simulink model "Fusion_Frame_Model_Architecture"  (R2018a)
settings: Solver=FixedStepAuto  StartTime=0.0  StopTime=SimulationTime  FixedStep=SamplingTime  RelTol=1e-3
undefined symbols (not defined in the file or in its folder): ACTIVATE_CAM, ACTIVATE_RAD, CAM1_detTimeStamp, CAM1_MeasNoise, CAM1_objClassID, CAM1_PX, CAM1_PY, CAM1_VX, CAM1_VY, CAM2_detTimeStamp, CAM2_MeasNoise, CAM2_objClassID, CAM2_PX, CAM2_PY, CAM2_VX, CAM2_VY, CAM3_detTimeStamp, CAM3_MeasNoise, CAM3_objClassID, CAM3_PX, CAM3_PY, CAM3_VX, CAM3_VY, CAM4_detTimeStamp, CAM4_MeasNoise, CAM4_objClassID, CAM4_PX, CAM4_PY, CAM4_VX, CAM4_VY, CAM5_detTimeStamp, CAM5_MeasNoise, CAM5_objClassID, CAM5_PX, CAM5_PY, CAM5_VX, CAM5_VY, CAM6_detTimeStamp, CAM6_MeasNoise, CAM6_objClassID, CAM6_PX, CAM6_PY, CAM6_VX, CAM6_VY, CAM7_detTimeStamp, CAM7_MeasNoise, CAM7_objClassID, CAM7_PX, CAM7_PY, CAM7_VX, CAM7_VY, CAM8_detTimeStamp, CAM8_MeasNoise, CAM8_objClassID, CAM8_PX, CAM8_PY, CAM8_VX, CAM8_VY, CAM_nMeas, CAM_TYPE ... (+181)
libraries: simulink_extras x4
(part 4 of 11)

== system Fusion_Frame_Model_Architecture/SENSOR_FUSION_SYSTEM/OBJECT_TRACKER_SENSOR_FUSION/SENSOR_LAYOUT_AND_CHRACTERIZATION/PRE_COMPUTE_SENSOR_FOV_GRID/SET_DATA ==
  GRID_PARAM : Inport
  RAD_REGION_CONFIDENCE : Inport  Port=2
  RAD_FOV_OVERLAP : Inport  Port=3
  CAM_REGION_CONFIDENCE : Inport  Port=4
  CAM_FOV_OVERLAP : Inport  Port=5
  Bus Creator : BusCreator  Inputs=2  OutDataTypeStr=Bus: RAD_GRID  NonVirtualBus=on
      settings: InheritFromInputs=off
  Bus Creator1 : BusCreator  Inputs=2  OutDataTypeStr=Bus: CAM_GRID  NonVirtualBus=on
      settings: InheritFromInputs=off
  Bus Creator2 : BusCreator  Inputs=3  OutDataTypeStr=Bus: GRID  NonVirtualBus=on
      settings: InheritFromInputs=off
  GRID_CHARACTERIZATION : Outport
  wires:
  Bus Creator/1 -> Bus Creator2/2  "RAD_GRID"
  CAM_REGION_CONFIDENCE/1 -> Bus Creator1/1  "CAM_REGION_CONFIDENCE"
  CAM_FOV_OVERLAP/1 -> Bus Creator1/2  "CAM_FOV_OVERLAP"
  Bus Creator1/1 -> Bus Creator2/3  "CAM_GRID"
  GRID_PARAM/1 -> Bus Creator2/1  "GRID_PARAM"
  RAD_REGION_CONFIDENCE/1 -> Bus Creator/1  "RAD_REGION_CONFIDENCE"
  RAD_FOV_OVERLAP/1 -> Bus Creator/2  "RAD_FOV_OVERLAP"
  Bus Creator2/1 -> GRID_CHARACTERIZATION/1

== system Fusion_Frame_Model_Architecture/SENSOR_FUSION_SYSTEM/OBJECT_TRACKER_SENSOR_FUSION/SENSOR_LAYOUT_AND_CHRACTERIZATION/SET_SENSOR_CALLIBRATION_PARAMETER/SET_CAMERA_SENSOR_PARAM ==
  CAMSnsrParam : Inport
  GET_DATA : Subsystem
  SET_CAMERA_EXTRINSIC_PARAM : Subsystem  TreatAsAtomicUnit=on
  SET_CAMERA_INTRINSIC_PARAM : Subsystem  TreatAsAtomicUnit=on
  SET_DATA : Subsystem
  CAMSnsrParamUpd : Outport
  wires:
  SET_DATA/1(CAMSnsrParamUpd) -> CAMSnsrParamUpd/1
  CAMSnsrParam/1 -> GET_DATA/1(CAMSnsrParam)
  GET_DATA/2(CameraExtrinsics) -> SET_CAMERA_EXTRINSIC_PARAM/1(CameraCalibParam)
  GET_DATA/1(CameraIntrinsics) -> SET_CAMERA_INTRINSIC_PARAM/1(CameraCalibParam)
  SET_CAMERA_INTRINSIC_PARAM/1(CameraCalibParamSet) -> SET_DATA/1(CameraIntrinsics)
  SET_CAMERA_EXTRINSIC_PARAM/1(CameraCalibParamSet) -> SET_DATA/2(CameraExtrinsics)

== system Fusion_Frame_Model_Architecture/SENSOR_FUSION_SYSTEM/OBJECT_TRACKER_SENSOR_FUSION/SENSOR_LAYOUT_AND_CHRACTERIZATION/SET_SENSOR_CALLIBRATION_PARAMETER/SET_RADAR_SENSOR_PARAM ==
  RADSnsrParam : Inport
  GET_DATA : Subsystem
  SET_DATA : Subsystem
  SET_RADAR_EXTRINSIC_PARAM : Subsystem  TreatAsAtomicUnit=on
  SET_RADAR_INTRINSIC_PARAM : Subsystem  TreatAsAtomicUnit=on
  RADSnsrParamUpd : Outport
  wires:
  RADSnsrParam/1 -> GET_DATA/1(RADSnsrParam)
  SET_DATA/1(RADSnsrParamUpd) -> RADSnsrParamUpd/1
  GET_DATA/2(<RadarExtrinsics>) -> SET_RADAR_EXTRINSIC_PARAM/1(RadarCalibParam)
  SET_RADAR_EXTRINSIC_PARAM/1(RadarCalibParamSet) -> SET_DATA/2(RadarExtrinsics)  "RadarIntrinsics"
  GET_DATA/1(<RadarIntrinsics>) -> SET_RADAR_INTRINSIC_PARAM/1(RadarCalibParam)
  SET_RADAR_INTRINSIC_PARAM/1(RadarCalibParamSet) -> SET_DATA/1(RadarIntrinsics)  "RadarExtrinsics"

== system Fusion_Frame_Model_Architecture/SENSOR_FUSION_SYSTEM/OBJECT_TRACKER_SENSOR_FUSION/SPATIAL_ALLIGNMENT1/CAMERA_MEASUREMENTS_SPATIAL_ALLIGNMENT/For Iterator Subsystem ==
  CameraCallibrationParam : Inport
  RadarStartingIdx : Inport  Port=2
  C1 : Inport  Port=3
  C2 : Inport  Port=4
  C3 : Inport  Port=5
  C4 : Inport  Port=6
  C5 : Inport  Port=7
  C6 : Inport  Port=8
  C7 : Inport  Port=9
  C8 : Inport  Port=10
  For Iterator : ForIterator  ResetStates=reset  IterationLimit=nCameras
  For Iterator Subsystem : Subsystem  TreatAsAtomicUnit=on
  InformationExtraction : Subsystem
  Subsystem : Subsystem
  MaxNoValidMeas : Outport
  CameraMeasTransformed : Outport  Port=2
  CameraMeasCOVTransformed : Outport  Port=3
  CameraMeasRef : Outport  Port=4
  wires:
  CameraCallibrationParam/1 -> InformationExtraction/1(CameraCallibration)
  C1/1 -> InformationExtraction/3(C1)
  C2/1 -> InformationExtraction/4(C2)
  C3/1 -> InformationExtraction/5(C3)
  C4/1 -> InformationExtraction/6(C4)
  C5/1 -> InformationExtraction/7(C5)
  C6/1 -> InformationExtraction/8(C6)
  InformationExtraction/1(CameraCalib) -> For Iterator Subsystem/1(CameraCalibration)
  InformationExtraction/2(nCameraMeas) -> For Iterator Subsystem/2(nMeas)
  InformationExtraction/3(CameraCANBus) -> For Iterator Subsystem/3(CameraCAN)
  RadarStartingIdx/1 -> InformationExtraction/11(StartingIndexes)
  Subsystem/1(nValidMeasVector) -> MaxNoValidMeas/1
  InformationExtraction/4(MeasStartingIdx) -> Subsystem/6(StartIdx)
  C7/1 -> InformationExtraction/9(C7)
  C8/1 -> InformationExtraction/10(C8)
  For Iterator/1 -> Subsystem/1(SnsrIndex), InformationExtraction/2(CameraID)
  For Iterator Subsystem/1(nValidMeas) -> Subsystem/2(nValidMeas)
  For Iterator Subsystem/2(CameraMeasUpd) -> Subsystem/3(CameraCTSMeas)
  For Iterator Subsystem/3(CameraMeasNoiseCovUpd) -> Subsystem/4(CameraCTSNoiseCOV)
  For Iterator Subsystem/4(CameraMeasRefUpd) -> Subsystem/5(CameraCTSRef)
  Subsystem/2(CTSMat) -> CameraMeasTransformed/1
  Subsystem/4(CTSMatRef) -> CameraMeasRef/1
  Subsystem/3(CTSMatNoiseCOV) -> CameraMeasCOVTransformed/1

== system Fusion_Frame_Model_Architecture/SENSOR_FUSION_SYSTEM/OBJECT_TRACKER_SENSOR_FUSION/SPATIAL_ALLIGNMENT1/CAMERA_MEASUREMENTS_SPATIAL_ALLIGNMENT/RadarMeasurementIndexes2 ==
  validMeasCount : Inport
  CTSmeasMAT : Inport  Port=2
  CTSCovMAT : Inport  Port=3
  CTSRefMAT : Inport  Port=4
  Add{,1..6} (7 alike) : Sum
  Assignment1 : Assignment  NumberOfDimensions=2  DiagnosticForDimensions=Warning  IndexOptions=Assign all,Starting index (dialog)  Indices=1,1  OutputSizes=1,1
  Assignment2 : Assignment  NumberOfDimensions=3  DiagnosticForDimensions=Warning  IndexOptions=Assign all,Assign all,Starting index (dialog)  Indices=1,1,1  OutputSizes=1,1,1
  Assignment3 : Assignment  NumberOfDimensions=2  DiagnosticForDimensions=Warning  IndexOptions=Assign all,Starting index (dialog)  Indices=1,1  OutputSizes=1,1
  Bus Creator1 : BusCreator  Inputs=5  OutDataTypeStr=Bus: CAM_MEAS_MAT_CTS  NonVirtualBus=on
      settings: InheritFromInputs=off
  FIND1 : Subsystem  TreatAsAtomicUnit=on
  Find Nonzero Elements1 : Find  Commented=on  NumberOfInputDimensions=3
  Mux1 : Mux  Inputs=8
  Reshape1 : Reshape  OutputDimensionality=Row vector (2-D)
  Selector : Selector  NumberOfDimensions=2  InputPortWidth=3  IndexOptions=Select all,Index vector (dialog)  Indices=1,1  OutputSizes=1,1
  Selector1 : Selector  NumberOfDimensions=2  InputPortWidth=3  IndexOptions=Select all,Index vector (dialog)  Indices=6,7  OutputSizes=1,1
  Selector11 : Selector  NumberOfDimensions=2  InputPortWidth=3  IndexOptions=Index vector (dialog),Select all  Indices=1,1  OutputSizes=1,1
  Selector12 : Selector  NumberOfDimensions=2  InputPortWidth=3  IndexOptions=Select all,Index vector (port)  Indices=1,1  OutputSizes=1,1
  Selector14 : Selector  NumberOfDimensions=2  InputPortWidth=3  IndexOptions=Select all,Index vector (port)  Indices=1,1  OutputSizes=1,1
  Selector15 : Selector  NumberOfDimensions=3  InputPortWidth=3  IndexOptions=Select all,Select all,Index vector (port)  Indices=1,1,1  OutputSizes=1,1,1
  Selector2 : Selector  NumberOfDimensions=2  InputPortWidth=3  IndexOptions=Select all,Index vector (dialog)  Indices=5,2  OutputSizes=1,1
  Selector3 : Selector  NumberOfDimensions=2  InputPortWidth=3  IndexOptions=Select all,Index vector (dialog)  Indices=5,3  OutputSizes=1,1
  Selector4 : Selector  NumberOfDimensions=2  InputPortWidth=3  IndexOptions=Select all,Index vector (dialog)  Indices=5,5  OutputSizes=1,1
  Selector5 : Selector  NumberOfDimensions=2  InputPortWidth=3  IndexOptions=Select all,Index vector (dialog)  Indices=6,6  OutputSizes=1,1
  Selector6 : Selector  NumberOfDimensions=2  InputPortWidth=3  IndexOptions=Select all,Index vector (dialog)  Indices=6,8  OutputSizes=1,1
  Selector8 : Selector  NumberOfDimensions=2  InputPortWidth=3  IndexOptions=Select all,Index vector (dialog)  Indices=5,4  OutputSizes=1,1
  CTSmeasMATout : Outport
  wires:
  validMeasCount/1 -> Selector2/1, Selector/1, Bus Creator1/4, Selector3/1, Selector6/1, Selector1/1, Selector5/1, Selector4/1, Selector8/1  "ValidMeasCountMeasCount"
  Add3/1 -> Add4/1, Mux1/5
  Selector3/1 -> Add1/2
  Add2/1 -> Add3/1, Mux1/4
  Add1/1 -> Mux1/3, Add2/1
  Selector4/1 -> Add3/2
  Selector/1 -> Mux1/1, Add/1
  Add/1 -> Add1/1, Mux1/2
  Add4/1 -> Add5/1, Mux1/6
  Selector2/1 -> Add/2
  Selector8/1 -> Add2/2
  Mux1/1 -> Reshape1/1
  Selector5/1 -> Add4/2
  Bus Creator1/1 -> CTSmeasMATout/1
  CTSRefMAT/1 -> [Ref], Selector11/1
  Selector11/1 -> FIND1/1(measIdx)
  FIND1/1(ValidIndex) -> Selector14/2, Selector12/2, Selector15/2
  CTSmeasMAT/1 -> Assignment1/1, Selector14/1
  Selector14/1 -> Assignment1/2
  Selector15/1 -> Assignment2/2
  Selector12/1 -> Assignment3/2
  CTSCovMAT/1 -> Assignment2/1, Selector15/1
  Assignment3/1 -> Bus Creator1/3  "MeasRef"
  Assignment2/1 -> Bus Creator1/2  "MeasCovariance"
  Assignment1/1 -> Bus Creator1/1  "MeasArray"
  [Ref] -> Assignment3/1, Selector12/1
  Reshape1/1 -> Bus Creator1/5  "ValidCumulativeMeasCount"
  Add5/1 -> Add6/1, Mux1/7
  Selector1/1 -> Add5/2
  Add6/1 -> Mux1/8
  Selector6/1 -> Add6/2

== system Fusion_Frame_Model_Architecture/SENSOR_FUSION_SYSTEM/OBJECT_TRACKER_SENSOR_FUSION/SPATIAL_ALLIGNMENT1/CAMERA_MEASUREMENTS_SPATIAL_ALLIGNMENT/StartingIndexes1 ==
  SnsrCallib : Inport
  CallibrationInfoExtractor : Subsystem
  Subsystem : Subsystem
  StartingIndexes : Outport
  wires:
  CallibrationInfoExtractor/1(C1nMeas) -> Subsystem/1(C1nMeas)
  CallibrationInfoExtractor/2(C2nMeas) -> Subsystem/2(C2nMeas)
  CallibrationInfoExtractor/3(C3nMeas) -> Subsystem/3(C3nMeas)
  CallibrationInfoExtractor/4(C4nMeas) -> Subsystem/4(C4nMeas)
  CallibrationInfoExtractor/5(C5nMeas) -> Subsystem/5(C5nMeas)
  Subsystem/1(StartingIndexes) -> StartingIndexes/1
  SnsrCallib/1 -> CallibrationInfoExtractor/1(SnsrCallib)
  CallibrationInfoExtractor/6(C6nMeas) -> Subsystem/6(C6nMeas)
  CallibrationInfoExtractor/7(C7nMeas) -> Subsystem/7(C7nMeas)

== system Fusion_Frame_Model_Architecture/SENSOR_FUSION_SYSTEM/OBJECT_TRACKER_SENSOR_FUSION/SPATIAL_ALLIGNMENT1/RADAR_MEASUREMENTS_SPATIAL_ALLIGNMENT/RADAR_MEASUREMENTS_SPATIAL_ALLIGNMENT ==
  RadarCallibrationParam : Inport
  RadarStartingIdx : Inport  Port=2
  R1 : Inport  Port=3
  R2 : Inport  Port=4
  R3 : Inport  Port=5
  R4 : Inport  Port=6
  R5 : Inport  Port=7
  R6 : Inport  Port=8
  COORDINATE_TRANSFORMATION : Subsystem  TreatAsAtomicUnit=on
  GET_DATA : Subsystem
  SENSOR_LOOP : ForIterator  ResetStates=reset  IterationLimit=nRadars
  SET_DATA : Subsystem
  RadarMeasTransformed : Outport
  RadarMeasCOVTransformed : Outport  Port=2
  RadarMeasRef : Outport  Port=3
  MaxNoValidMeas : Outport  Port=4
  wires:
  RadarCallibrationParam/1 -> GET_DATA/1(RadarCallibration)
  R1/1 -> GET_DATA/3(R1)
  R2/1 -> GET_DATA/4(R2)
  R3/1 -> GET_DATA/5(R3)
  R4/1 -> GET_DATA/6(R4)
  R5/1 -> GET_DATA/7(R5)
  R6/1 -> GET_DATA/8(R6)
  GET_DATA/1(RadarCalib) -> COORDINATE_TRANSFORMATION/1(RadarCalibration)
  GET_DATA/2(nRadarMeas) -> COORDINATE_TRANSFORMATION/2(nMeas)
  GET_DATA/3(RadarCANBus) -> COORDINATE_TRANSFORMATION/3(RadarCAN)
  RadarStartingIdx/1 -> GET_DATA/9(StartingIndexes)
  SENSOR_LOOP/1 -> SET_DATA/1(SnsrIndex), GET_DATA/2(RadarID)
  SET_DATA/1(nValidMeasVector) -> MaxNoValidMeas/1
  GET_DATA/4(MeasStartingIdx) -> SET_DATA/6(StartIdx)
  COORDINATE_TRANSFORMATION/1(nValidMeas) -> SET_DATA/2(nValidMeas)
  COORDINATE_TRANSFORMATION/2(RadarMeasUpd) -> SET_DATA/3(RadarCTSMeas)
  SET_DATA/2(CTSMat) -> RadarMeasTransformed/1
  COORDINATE_TRANSFORMATION/3(RadarMeasNoiseCovUpd) -> SET_DATA/4(RadarCTSNoiseCOV)
  COORDINATE_TRANSFORMATION/4(RadarMeasRefUpd) -> SET_DATA/5(RadarCTSRef)
  SET_DATA/4(CTSMatRef) -> RadarMeasRef/1
  SET_DATA/3(CTSMatNoiseCOV) -> RadarMeasCOVTransformed/1

== system Fusion_Frame_Model_Architecture/SENSOR_FUSION_SYSTEM/OBJECT_TRACKER_SENSOR_FUSION/SPATIAL_ALLIGNMENT1/RADAR_MEASUREMENTS_SPATIAL_ALLIGNMENT/SET_MEASUREMENTS ==
  CTSmeasMAT : Inport
  CTSCovMAT : Inport  Port=2
  CTSRefMAT : Inport  Port=3
  validMeasCount : Inport  Port=4
  Add{,1..4} (5 alike) : Sum
  Assignment1 : Assignment  NumberOfDimensions=2  DiagnosticForDimensions=Warning  IndexOptions=Assign all,Starting index (dialog)  Indices=1,1  OutputSizes=1,1
  Assignment2 : Assignment  NumberOfDimensions=3  DiagnosticForDimensions=Warning  IndexOptions=Assign all,Assign all,Starting index (dialog)  Indices=1,1,1  OutputSizes=1,1,1
  Assignment3 : Assignment  NumberOfDimensions=2  DiagnosticForDimensions=Warning  IndexOptions=Assign all,Starting index (dialog)  Indices=1,1  OutputSizes=1,1
  Bus Creator1 : BusCreator  Inputs=5  OutDataTypeStr=Bus: RAD_MEAS_MAT_CTS  NonVirtualBus=on
      settings: InheritFromInputs=off
  FIND : Subsystem  TreatAsAtomicUnit=on
  Find Nonzero Elements1 : Find  Commented=on  NumberOfInputDimensions=3
  Mux1 : Mux  Inputs=6
  Reshape1 : Reshape  OutputDimensionality=Row vector (2-D)
  Selector : Selector  NumberOfDimensions=2  InputPortWidth=3  IndexOptions=Select all,Index vector (dialog)  Indices=1,1  OutputSizes=1,1
  Selector11 : Selector  NumberOfDimensions=2  InputPortWidth=3  IndexOptions=Index vector (dialog),Select all  Indices=1,1  OutputSizes=1,1
  Selector12 : Selector  NumberOfDimensions=2  InputPortWidth=3  IndexOptions=Select all,Index vector (port)  Indices=1,1  OutputSizes=1,1
  Selector14 : Selector  NumberOfDimensions=2  InputPortWidth=3  IndexOptions=Select all,Index vector (port)  Indices=1,1  OutputSizes=1,1
  Selector15 : Selector  NumberOfDimensions=3  InputPortWidth=3  IndexOptions=Select all,Select all,Index vector (port)  Indices=1,1,1  OutputSizes=1,1,1
  Selector2 : Selector  NumberOfDimensions=2  InputPortWidth=3  IndexOptions=Select all,Index vector (dialog)  Indices=5,2  OutputSizes=1,1
  Selector3 : Selector  NumberOfDimensions=2  InputPortWidth=3  IndexOptions=Select all,Index vector (dialog)  Indices=5,3  OutputSizes=1,1
  Selector4 : Selector  NumberOfDimensions=2  InputPortWidth=3  IndexOptions=Select all,Index vector (dialog)  Indices=5,5  OutputSizes=1,1
  Selector5 : Selector  NumberOfDimensions=2  InputPortWidth=3  IndexOptions=Select all,Index vector (dialog)  Indices=6,6  OutputSizes=1,1
  Selector8 : Selector  NumberOfDimensions=2  InputPortWidth=3  IndexOptions=Select all,Index vector (dialog)  Indices=5,4  OutputSizes=1,1
  CTSmeasMATout : Outport
  wires:
  validMeasCount/1 -> Selector2/1, Selector/1, Bus Creator1/4, Selector3/1, Selector8/1, Selector4/1, Selector5/1  "ValidMeasCountMeasCount"
  Add3/1 -> Add4/1, Mux1/5
  Selector3/1 -> Add1/2
  Add2/1 -> Add3/1, Mux1/4
  Add1/1 -> Mux1/3, Add2/1
  Selector4/1 -> Add3/2
  Selector/1 -> Mux1/1, Add/1
  Add/1 -> Add1/1, Mux1/2
  Add4/1 -> Mux1/6
  Selector2/1 -> Add/2
  Selector8/1 -> Add2/2
  Mux1/1 -> Reshape1/1
  Selector5/1 -> Add4/2
  Bus Creator1/1 -> CTSmeasMATout/1
  CTSRefMAT/1 -> [Ref], Selector11/1
  Selector11/1 -> FIND/1(measIdx)
  FIND/1(ValidIndex) -> Selector14/2, Selector12/2, Selector15/2
  CTSmeasMAT/1 -> Assignment1/1, Selector14/1
  Selector14/1 -> Assignment1/2
  Selector15/1 -> Assignment2/2
  Selector12/1 -> Assignment3/2
  CTSCovMAT/1 -> Assignment2/1, Selector15/1
  Assignment3/1 -> Bus Creator1/3  "MeasRef"
  Assignment2/1 -> Bus Creator1/2  "MeasCovariance"
  Assignment1/1 -> Bus Creator1/1  "MeasArray"
  [Ref] -> Assignment3/1, Selector12/1
  Reshape1/1 -> Bus Creator1/5  "ValidCumulativeMeasCount"

== system Fusion_Frame_Model_Architecture/SENSOR_FUSION_SYSTEM/OBJECT_TRACKER_SENSOR_FUSION/SPATIAL_ALLIGNMENT1/RADAR_MEASUREMENTS_SPATIAL_ALLIGNMENT/StartingIndexes1 ==
  SnsrCallib : Inport
  CallibrationInfoExtractor : Subsystem
  Subsystem : Subsystem
  StartingIndexes : Outport
  wires:
  CallibrationInfoExtractor/1(R1nMeas) -> Subsystem/1(R1nMeas)
  CallibrationInfoExtractor/2(R2nMeas) -> Subsystem/2(R2nMeas)
  CallibrationInfoExtractor/3(R3nMeas) -> Subsystem/3(R3nMeas)
  CallibrationInfoExtractor/4(R4nMeas) -> Subsystem/4(R4nMeas)
  CallibrationInfoExtractor/5(R5nMeas) -> Subsystem/5(R5nMeas)
  Subsystem/1(StartingIndexes) -> StartingIndexes/1
  SnsrCallib/1 -> CallibrationInfoExtractor/1(SnsrCallib)

== system Fusion_Frame_Model_Architecture/SENSOR_FUSION_SYSTEM/ROAD_GEOMETRY_CAMERA_FUSION/ROAD_GEOMERY_AND_GRID_COMPUTATION/COMPUTE_LEFT_LINE/CURVE_FITTING_BY_LEAST_SQUARES ==
  Points : Inport
  Ground : Ground
  Terminator : Terminator
  PolynomialCoefficients : Outport
  wires:
  Points/1 -> Terminator/1
  Ground/1 -> PolynomialCoefficients/1

== system Fusion_Frame_Model_Architecture/SENSOR_FUSION_SYSTEM/ROAD_GEOMETRY_CAMERA_FUSION/ROAD_GEOMERY_AND_GRID_COMPUTATION/COMPUTE_LEFT_LINE/GENERATE_POINTS_ON_THE_LANE_BORDER ==
  PointsAlongTheLine : Inport
  EgoLaneWidth : Inport  Port=2
  Ground : Ground
  Terminator : Terminator
  Terminator1 : Terminator
  PointsAlongTheLinea : Outport
  wires:
  Ground/1 -> PointsAlongTheLinea/1
  EgoLaneWidth/1 -> Terminator1/1
  PointsAlongTheLine/1 -> Terminator/1

== system Fusion_Frame_Model_Architecture/SENSOR_FUSION_SYSTEM/ROAD_GEOMETRY_CAMERA_FUSION/ROAD_GEOMERY_AND_GRID_COMPUTATION/COMPUTE_LEFT_LINE/INTERPOLATE_POINTS_ALONG_THE_EGO_LANE_CENTER_LINE ==
  EGO_LANE_CENTER_LINE_TRACK : Inport
  Ground : Ground
  Terminator : Terminator
  PointsAlongTheLine : Outport
  wires:
  EGO_LANE_CENTER_LINE_TRACK/1 -> Terminator/1
  Ground/1 -> PointsAlongTheLine/1

== system Fusion_Frame_Model_Architecture/SENSOR_FUSION_SYSTEM/ROAD_GEOMETRY_CAMERA_FUSION/ROAD_GEOMERY_AND_GRID_COMPUTATION/COMPUTE_LEFT_LINE/POLYNOMIAL_TO_CLOTHOID_CONVERSION ==
  PolynomialCoefficients : Inport
  Ground : Ground
  Terminator : Terminator
  ClothoidCoefficients : Outport  OutDataTypeStr=Bus: ClothoidParamBus
  wires:
  PolynomialCoefficients/1 -> Terminator/1
  Ground/1 -> ClothoidCoefficients/1

== system Fusion_Frame_Model_Architecture/SENSOR_FUSION_SYSTEM/ROAD_GEOMETRY_CAMERA_FUSION/ROAD_GEOMERY_AND_GRID_COMPUTATION/COMPUTE_NEXT_LEFT_LINE/CURVE_FITTING_BY_LEAST_SQUARES ==
  Points : Inport
  Ground : Ground
  Terminator : Terminator
  PolynomialCoefficients : Outport
  wires:
  Points/1 -> Terminator/1
  Ground/1 -> PolynomialCoefficients/1

== system Fusion_Frame_Model_Architecture/SENSOR_FUSION_SYSTEM/ROAD_GEOMETRY_CAMERA_FUSION/ROAD_GEOMERY_AND_GRID_COMPUTATION/COMPUTE_NEXT_LEFT_LINE/GENERATE_POINTS_ON_THE_LANE_BORDER ==
  PointsAlongTheLine : Inport
  EgoLaneWidth : Inport  Port=2
  Ground : Ground
  Terminator : Terminator
  Terminator1 : Terminator
  PointsAlongTheLinea : Outport
  wires:
  Ground/1 -> PointsAlongTheLinea/1
  EgoLaneWidth/1 -> Terminator1/1
  PointsAlongTheLine/1 -> Terminator/1

== system Fusion_Frame_Model_Architecture/SENSOR_FUSION_SYSTEM/ROAD_GEOMETRY_CAMERA_FUSION/ROAD_GEOMERY_AND_GRID_COMPUTATION/COMPUTE_NEXT_LEFT_LINE/INTERPOLATE_POINTS_ALONG_THE_EGO_LANE_CENTER_LINE ==
  EGO_LANE_CENTER_LINE_TRACK : Inport
  Ground : Ground
  Terminator : Terminator
  PointsAlongTheLine : Outport
  wires:
  EGO_LANE_CENTER_LINE_TRACK/1 -> Terminator/1
  Ground/1 -> PointsAlongTheLine/1

== system Fusion_Frame_Model_Architecture/SENSOR_FUSION_SYSTEM/ROAD_GEOMETRY_CAMERA_FUSION/ROAD_GEOMERY_AND_GRID_COMPUTATION/COMPUTE_NEXT_LEFT_LINE/POLYNOMIAL_TO_CLOTHOID_CONVERSION ==
  PolynomialCoefficients : Inport
  Ground : Ground
  Terminator : Terminator
  ClothoidCoefficients : Outport  OutDataTypeStr=Bus: ClothoidParamBus
  wires:
  PolynomialCoefficients/1 -> Terminator/1
  Ground/1 -> ClothoidCoefficients/1

== system Fusion_Frame_Model_Architecture/SENSOR_FUSION_SYSTEM/ROAD_GEOMETRY_CAMERA_FUSION/ROAD_GEOMERY_AND_GRID_COMPUTATION/COMPUTE_NEXT_NEXT_LEFT_LINE/CURVE_FITTING_BY_LEAST_SQUARES ==
  Points : Inport
  Ground : Ground
  Terminator : Terminator
  PolynomialCoefficients : Outport
  wires:
  Points/1 -> Terminator/1
  Ground/1 -> PolynomialCoefficients/1

== system Fusion_Frame_Model_Architecture/SENSOR_FUSION_SYSTEM/ROAD_GEOMETRY_CAMERA_FUSION/ROAD_GEOMERY_AND_GRID_COMPUTATION/COMPUTE_NEXT_NEXT_LEFT_LINE/GENERATE_POINTS_ON_THE_LANE_BORDER ==
  PointsAlongTheLine : Inport
  EgoLaneWidth : Inport  Port=2
  Ground : Ground
  Terminator : Terminator
  Terminator1 : Terminator
  PointsAlongTheLinea : Outport
  wires:
  Ground/1 -> PointsAlongTheLinea/1
  EgoLaneWidth/1 -> Terminator1/1
  PointsAlongTheLine/1 -> Terminator/1

== system Fusion_Frame_Model_Architecture/SENSOR_FUSION_SYSTEM/ROAD_GEOMETRY_CAMERA_FUSION/ROAD_GEOMERY_AND_GRID_COMPUTATION/COMPUTE_NEXT_NEXT_LEFT_LINE/INTERPOLATE_POINTS_ALONG_THE_EGO_LANE_CENTER_LINE ==
  EGO_LANE_CENTER_LINE_TRACK : Inport
  Ground : Ground
  Terminator : Terminator
  PointsAlongTheLine : Outport
  wires:
  EGO_LANE_CENTER_LINE_TRACK/1 -> Terminator/1
  Ground/1 -> PointsAlongTheLine/1

== system Fusion_Frame_Model_Architecture/SENSOR_FUSION_SYSTEM/ROAD_GEOMETRY_CAMERA_FUSION/ROAD_GEOMERY_AND_GRID_COMPUTATION/COMPUTE_NEXT_NEXT_LEFT_LINE/POLYNOMIAL_TO_CLOTHOID_CONVERSION ==
  PolynomialCoefficients : Inport
  Ground : Ground
  Terminator : Terminator
  ClothoidCoefficients : Outport  OutDataTypeStr=Bus: ClothoidParamBus
  wires:
  PolynomialCoefficients/1 -> Terminator/1
  Ground/1 -> ClothoidCoefficients/1

== system Fusion_Frame_Model_Architecture/SENSOR_FUSION_SYSTEM/ROAD_GEOMETRY_CAMERA_FUSION/ROAD_GEOMERY_AND_GRID_COMPUTATION/COMPUTE_NEXT_NEXT_RIGHT_LINE/CURVE_FITTING_BY_LEAST_SQUARES ==
  Points : Inport
  Ground : Ground
  Terminator : Terminator
  PolynomialCoefficients : Outport
  wires:
  Points/1 -> Terminator/1
  Ground/1 -> PolynomialCoefficients/1

== system Fusion_Frame_Model_Architecture/SENSOR_FUSION_SYSTEM/ROAD_GEOMETRY_CAMERA_FUSION/ROAD_GEOMERY_AND_GRID_COMPUTATION/COMPUTE_NEXT_NEXT_RIGHT_LINE/GENERATE_POINTS_ON_THE_LANE_BORDER ==
  PointsAlongTheLine : Inport
  EgoLaneWidth : Inport  Port=2
  Ground : Ground
  Terminator : Terminator
  Terminator1 : Terminator
  PointsAlongTheLinea : Outport
  wires:
  Ground/1 -> PointsAlongTheLinea/1
  EgoLaneWidth/1 -> Terminator1/1
  PointsAlongTheLine/1 -> Terminator/1

== system Fusion_Frame_Model_Architecture/SENSOR_FUSION_SYSTEM/ROAD_GEOMETRY_CAMERA_FUSION/ROAD_GEOMERY_AND_GRID_COMPUTATION/COMPUTE_NEXT_NEXT_RIGHT_LINE/INTERPOLATE_POINTS_ALONG_THE_EGO_LANE_CENTER_LINE ==
  EGO_LANE_CENTER_LINE_TRACK : Inport
  Ground : Ground
  Terminator : Terminator
  PointsAlongTheLine : Outport
  wires:
  EGO_LANE_CENTER_LINE_TRACK/1 -> Terminator/1
  Ground/1 -> PointsAlongTheLine/1

== system Fusion_Frame_Model_Architecture/SENSOR_FUSION_SYSTEM/ROAD_GEOMETRY_CAMERA_FUSION/ROAD_GEOMERY_AND_GRID_COMPUTATION/COMPUTE_NEXT_NEXT_RIGHT_LINE/POLYNOMIAL_TO_CLOTHOID_CONVERSION ==
  PolynomialCoefficients : Inport
  Ground : Ground
  Terminator : Terminator
  ClothoidCoefficients : Outport  OutDataTypeStr=Bus: ClothoidParamBus
  wires:
  PolynomialCoefficients/1 -> Terminator/1
  Ground/1 -> ClothoidCoefficients/1

== system Fusion_Frame_Model_Architecture/SENSOR_FUSION_SYSTEM/ROAD_GEOMETRY_CAMERA_FUSION/ROAD_GEOMERY_AND_GRID_COMPUTATION/COMPUTE_NEXT_RIGHT_LINE/CURVE_FITTING_BY_LEAST_SQUARES ==
  Points : Inport
  Ground : Ground
  Terminator : Terminator
  PolynomialCoefficients : Outport
  wires:
  Points/1 -> Terminator/1
  Ground/1 -> PolynomialCoefficients/1

== system Fusion_Frame_Model_Architecture/SENSOR_FUSION_SYSTEM/ROAD_GEOMETRY_CAMERA_FUSION/ROAD_GEOMERY_AND_GRID_COMPUTATION/COMPUTE_NEXT_RIGHT_LINE/GENERATE_POINTS_ON_THE_LANE_BORDER ==
  PointsAlongTheLine : Inport
  EgoLaneWidth : Inport  Port=2
  Ground : Ground
  Terminator : Terminator
  Terminator1 : Terminator
  PointsAlongTheLinea : Outport
  wires:
  Ground/1 -> PointsAlongTheLinea/1
  EgoLaneWidth/1 -> Terminator1/1
  PointsAlongTheLine/1 -> Terminator/1

== system Fusion_Frame_Model_Architecture/SENSOR_FUSION_SYSTEM/ROAD_GEOMETRY_CAMERA_FUSION/ROAD_GEOMERY_AND_GRID_COMPUTATION/COMPUTE_NEXT_RIGHT_LINE/INTERPOLATE_POINTS_ALONG_THE_EGO_LANE_CENTER_LINE ==
  EGO_LANE_CENTER_LINE_TRACK : Inport
  Ground : Ground
  Terminator : Terminator
  PointsAlongTheLine : Outport
  wires:
  EGO_LANE_CENTER_LINE_TRACK/1 -> Terminator/1
  Ground/1 -> PointsAlongTheLine/1

== system Fusion_Frame_Model_Architecture/SENSOR_FUSION_SYSTEM/ROAD_GEOMETRY_CAMERA_FUSION/ROAD_GEOMERY_AND_GRID_COMPUTATION/COMPUTE_NEXT_RIGHT_LINE/POLYNOMIAL_TO_CLOTHOID_CONVERSION ==
  PolynomialCoefficients : Inport
  Ground : Ground
  Terminator : Terminator
  ClothoidCoefficients : Outport  OutDataTypeStr=Bus: ClothoidParamBus
  wires:
  PolynomialCoefficients/1 -> Terminator/1
  Ground/1 -> ClothoidCoefficients/1

== system Fusion_Frame_Model_Architecture/SENSOR_FUSION_SYSTEM/ROAD_GEOMETRY_CAMERA_FUSION/ROAD_GEOMERY_AND_GRID_COMPUTATION/COMPUTE_RIGHT_LINE/CURVE_FITTING_BY_LEAST_SQUARES ==
  Points : Inport
  Ground : Ground
  Terminator : Terminator
  PolynomialCoefficients : Outport
  wires:
  Points/1 -> Terminator/1
  Ground/1 -> PolynomialCoefficients/1

== system Fusion_Frame_Model_Architecture/SENSOR_FUSION_SYSTEM/ROAD_GEOMETRY_CAMERA_FUSION/ROAD_GEOMERY_AND_GRID_COMPUTATION/COMPUTE_RIGHT_LINE/GENERATE_POINTS_ON_THE_LANE_BORDER ==
  PointsAlongTheLine : Inport
  EgoLaneWidth : Inport  Port=2
  Ground : Ground
  Terminator : Terminator
  Terminator1 : Terminator
  PointsAlongTheLinea : Outport
  wires:
  Ground/1 -> PointsAlongTheLinea/1
  EgoLaneWidth/1 -> Terminator1/1
  PointsAlongTheLine/1 -> Terminator/1

== system Fusion_Frame_Model_Architecture/SENSOR_FUSION_SYSTEM/ROAD_GEOMETRY_CAMERA_FUSION/ROAD_GEOMERY_AND_GRID_COMPUTATION/COMPUTE_RIGHT_LINE/INTERPOLATE_POINTS_ALONG_THE_EGO_LANE_CENTER_LINE ==
  EGO_LANE_CENTER_LINE_TRACK : Inport
  Ground : Ground
  Terminator : Terminator
  PointsAlongTheLine : Outport
  wires:
  EGO_LANE_CENTER_LINE_TRACK/1 -> Terminator/1
  Ground/1 -> PointsAlongTheLine/1

== system Fusion_Frame_Model_Architecture/SENSOR_FUSION_SYSTEM/ROAD_GEOMETRY_CAMERA_FUSION/ROAD_GEOMERY_AND_GRID_COMPUTATION/COMPUTE_RIGHT_LINE/POLYNOMIAL_TO_CLOTHOID_CONVERSION ==
  PolynomialCoefficients : Inport
  Ground : Ground
  Terminator : Terminator
  ClothoidCoefficients : Outport  OutDataTypeStr=Bus: ClothoidParamBus
  wires:
  PolynomialCoefficients/1 -> Terminator/1
  Ground/1 -> ClothoidCoefficients/1

== system Fusion_Frame_Model_Architecture/SENSOR_FUSION_SYSTEM/ROAD_GEOMETRY_CAMERA_FUSION/ROAD_GEOMERY_AND_GRID_COMPUTATION/COMPUTE_ROAD_GRID/DISTANCE_TRAVELLED_BY_EGO_VEHICLE_DURING_DT ==
  EgoParam : Inport
  Ground : Ground
  Ground1 : Ground
  Ground2 : Ground
  Terminator : Terminator
  dYaw : Outport
  dX : Outport  Port=2
  dY : Outport  Port=3
  wires:
  EgoParam/1 -> Terminator/1
  Ground/1 -> dYaw/1
  Ground1/1 -> dX/1
  Ground2/1 -> dY/1

== system Fusion_Frame_Model_Architecture/SENSOR_FUSION_SYSTEM/ROAD_GEOMETRY_CAMERA_FUSION/ROAD_GEOMERY_AND_GRID_COMPUTATION/COMPUTE_ROAD_GRID/EGO_COMPENSATION_FOR_ROAD_GRID_PREDICTION ==
  ROAD_GRID_prev : Inport
  dYaw : Inport  Port=2
  dX : Inport  Port=3
  dY : Inport  Port=4
  Terminator : Terminator
  Terminator1 : Terminator
  Terminator2 : Terminator
  Unit Delay : UnitDelay  InitialCondition=ROAD_GRID_STRUCT  SampleTime=-1
  ROAD_GRID_egoCompensated : Outport
  wires:
  ROAD_GRID_prev/1 -> Unit Delay/1
  Unit Delay/1 -> ROAD_GRID_egoCompensated/1
  dYaw/1 -> Terminator/1
  dX/1 -> Terminator1/1
  dY/1 -> Terminator2/1

== system Fusion_Frame_Model_Architecture/SENSOR_FUSION_SYSTEM/ROAD_GEOMETRY_CAMERA_FUSION/ROAD_GEOMERY_AND_GRID_COMPUTATION/COMPUTE_ROAD_GRID/ROAD_GRID_UPDATE ==
  ROAD_GRID_Pred : Inport
  RPAD_GEOMETRY : Inport  Port=2
  Bus Creator : BusCreator  Inputs=7  OutDataTypeStr=Bus: ROAD_GRID  NonVirtualBus=on
      settings: InheritFromInputs=off
  Bus Selector : BusSelector  OutputSignals=EgoLaneNxtNxtLeftBoundary,EgoLaneNxtLeftBoundary,EgoLaneLeftBoundary,EgoLaneCenter,EgoLaneRightBoundary,EgoLaneNxtRightBoundary,EgoLaneNxtNxtRightBoundary
  Terminator : Terminator
  ROAD_GRID_Upd : Outport
  wires:
  RPAD_GEOMETRY/1 -> Terminator/1
  ROAD_GRID_Pred/1 -> Bus Selector/1
  Bus Selector/1 -> Bus Creator/1  "<EgoLaneNxtNxtLeftBoundary>"
  Bus Selector/2 -> Bus Creator/2  "<EgoLaneNxtLeftBoundary>"
  Bus Selector/3 -> Bus Creator/3  "<EgoLaneLeftBoundary>"
  Bus Selector/4 -> Bus Creator/4  "<EgoLaneCenter>"
  Bus Selector/5 -> Bus Creator/5  "<EgoLaneRightBoundary>"
  Bus Selector/6 -> Bus Creator/6  "<EgoLaneNxtRightBoundary>"
  Bus Selector/7 -> Bus Creator/7  "<EgoLaneNxtNxtRightBoundary>"
  Bus Creator/1 -> ROAD_GRID_Upd/1

== system Fusion_Frame_Model_Architecture/SENSOR_MEASUREMENTS/RADAR_CAMERA_EGO_SENSOR_INTERFACE/CameraSensors/Camera1/CHECK_IF_DATA_IS_VALID ==
  idx : Inport
  px : Inport  Port=2
  py : Inport  Port=3
  vx : Inport  Port=4
  vy : Inport  Port=5
  Abs{,1..3} (4 alike) : Abs
  Add : Sum  Inputs=++++
  Constant : Constant  Value=uint16(0)
  Data Type Conversion : DataTypeConversion  OutDataTypeStr=uint16
  Switch : Switch  Threshold=0.0001
  ID : Outport
  wires:
  Add/1 -> Switch/2
  Abs2/1 -> Add/3
  Constant/1 -> Switch/3
  Abs/1 -> Add/1
  px/1 -> Abs/1
  Abs3/1 -> Add/4
  Abs1/1 -> Add/2
  vy/1 -> Abs3/1
  py/1 -> Abs1/1
  vx/1 -> Abs2/1
  idx/1 -> Data Type Conversion/1
  Switch/1 -> ID/1
  Data Type Conversion/1 -> Switch/1

== system Fusion_Frame_Model_Architecture/SENSOR_MEASUREMENTS/RADAR_CAMERA_EGO_SENSOR_INTERFACE/CameraSensors/Camera1/GET_DATA ==
  idx : Inport
  time : Inport  Port=2
  Constant : Constant  Value=CAM1_PX
  Constant1 : Constant  Value=CAM1_PY
  Constant2 : Constant  Value=CAM1_VX
  Constant3 : Constant  Value=CAM1_VY
  Constant4 : Constant  Value=CAM1_objClassID
  Constant5 : Constant  Value=CAM1_MeasNoise
  Constant6 : Constant  Value=CAM1_detTimeStamp
  Data Type Conversion : DataTypeConversion  OutDataTypeStr=int16
  MeasNoise : Selector  NumberOfDimensions=4  InputPortWidth=3  IndexOptions=Index vector (port),Select all,Select all,Index vector (port)  Indices=[1 3],1,1,1  OutputSizes=1,1,1,1
  ObjectClass : Selector  NumberOfDimensions=2  InputPortWidth=3  IndexOptions=Index vector (port),Index vector (port)  Indices=[1 3],1  OutputSizes=1,1
  PosX : Selector  NumberOfDimensions=2  InputPortWidth=3  IndexOptions=Index vector (port),Index vector (port)  Indices=[1 3],1  OutputSizes=1,1
  PosY : Selector  NumberOfDimensions=2  InputPortWidth=3  IndexOptions=Index vector (port),Index vector (port)  Indices=[1 3],1  OutputSizes=1,1
  Reshape : Reshape  OutputDimensionality=Customize  OutputDimensions=[4,4]
  VelX : Selector  NumberOfDimensions=2  InputPortWidth=3  IndexOptions=Index vector (port),Index vector (port)  Indices=[1 3],1  OutputSizes=1,1
  VelY : Selector  NumberOfDimensions=2  InputPortWidth=3  IndexOptions=Index vector (port),Index vector (port)  Indices=[1 3],1  OutputSizes=1,1
  timeStamp : Selector  NumberOfDimensions=2  InputPortWidth=3  IndexOptions=Select all,Index vector (port)  Indices=[1 3],1  OutputSizes=1,1
  PX : Outport
  PY : Outport  Port=2
  VX : Outport  Port=3
  VY : Outport  Port=4
  OBJ_TYPE : Outport  Port=5
  NOISE_COV : Outport  Port=6
  measCaptureTime : Outport  Port=7
  wires:
  Constant3/1 -> VelY/1
  Constant2/1 -> VelX/1
  VelY/1 -> VY/1
  Constant/1 -> PosX/1
  idx/1 -> MeasNoise/3, ObjectClass/3, VelY/3, VelX/3, PosY/3, PosX/3
  Constant1/1 -> PosY/1
  VelX/1 -> VX/1
  PosX/1 -> PX/1
  PosY/1 -> PY/1
  time/1 -> timeStamp/2, MeasNoise/2, ObjectClass/2, VelY/2, VelX/2, PosY/2, PosX/2
  Constant4/1 -> ObjectClass/1
  ObjectClass/1 -> Data Type Conversion/1
  Constant5/1 -> MeasNoise/1
  Constant6/1 -> timeStamp/1
  MeasNoise/1 -> Reshape/1
  timeStamp/1 -> measCaptureTime/1
  Reshape/1 -> NOISE_COV/1
  Data Type Conversion/1 -> OBJ_TYPE/1

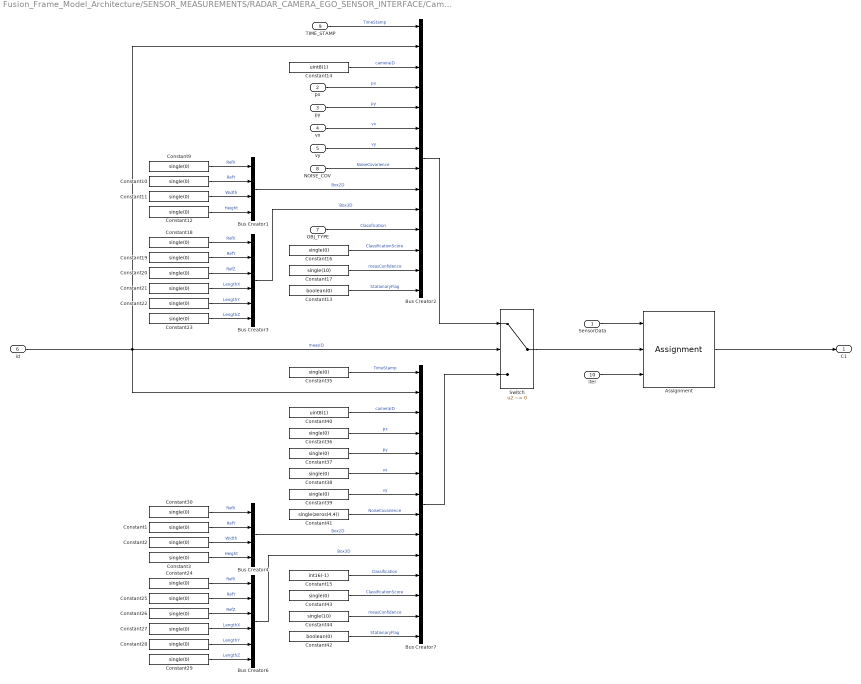
== system Fusion_Frame_Model_Architecture/SENSOR_MEASUREMENTS/RADAR_CAMERA_EGO_SENSOR_INTERFACE/CameraSensors/Camera1/SET_DATA ==
  SensorData : Inport
  px : Inport  Port=2
  py : Inport  Port=3
  vx : Inport  Port=4
  vy : Inport  Port=5
  id : Inport  Port=6
  OBJ_TYPE : Inport  Port=7
  NOISE_COV : Inport  Port=8
  TIME_STAMP : Inport  Port=9
  iter : Inport  Port=10
  Assignment : Assignment  DiagnosticForDimensions=Warning  IndexOptions=Index vector (port)  Indices=1  OutputSizes=1
  Bus Creator1 : BusCreator  Inputs=4  OutDataTypeStr=Bus: BoxParam2D  NonVirtualBus=on
  Bus Creator2 : BusCreator  Inputs=14  OutDataTypeStr=Bus: CameraMeasParam  NonVirtualBus=on
  Bus Creator3 : BusCreator  Inputs=6  OutDataTypeStr=Bus: BoxParam3D  NonVirtualBus=on
  Bus Creator4 : BusCreator  Inputs=4  OutDataTypeStr=Bus: BoxParam2D  NonVirtualBus=on
  Bus Creator6 : BusCreator  Inputs=6  OutDataTypeStr=Bus: BoxParam3D  NonVirtualBus=on
  Bus Creator7 : BusCreator  Inputs=14  OutDataTypeStr=Bus: CameraMeasParam  NonVirtualBus=on
  Constant{1..3,9..12,16,18..30,35..39,43} (27 alike) : Constant  Value=single(0)
  Constant13 : Constant  Value=boolean(0)
  Constant14 : Constant  Value=uint8(1)
  Constant15 : Constant  Value=int16(-1)
  Constant17 : Constant  Value=single(10)
  Constant40 : Constant  Value=uint8(1)
  Constant41 : Constant  Value=single(zeros(4,4))
  Constant42 : Constant  Value=boolean(0)
  Constant44 : Constant  Value=single(10)
  Switch : Switch  Criteria=u2 ~= 0
  C1 : Outport
  wires:
  Bus Creator4/1 -> Bus Creator7/9  "Box2D"
  Bus Creator1/1 -> Bus Creator2/9  "Box2D"
  Bus Creator7/1 -> Switch/3
  Constant3/1 -> Bus Creator4/4  "Height"
  Constant44/1 -> Bus Creator7/13  "measConfidence"
  Constant19/1 -> Bus Creator3/2  "RefY"
  id/1 -> Bus Creator7/2, Bus Creator2/2, Switch/2  "measID"
  Bus Creator2/1 -> Switch/1
  Constant2/1 -> Bus Creator4/3  "Width"
  Constant12/1 -> Bus Creator1/4  "Height"
  Constant43/1 -> Bus Creator7/12  "ClassificationScore"
  Constant41/1 -> Bus Creator7/8  "NoiseCovarience"
  Constant20/1 -> Bus Creator3/3  "RefZ"
  Constant37/1 -> Bus Creator7/5  "py"
  Constant23/1 -> Bus Creator3/6  "LengthZ"
  Constant11/1 -> Bus Creator1/3  "Width"
  Constant18/1 -> Bus Creator3/1  "RefX"
  Constant9/1 -> Bus Creator1/1  "RefX"
  Constant27/1 -> Bus Creator6/4  "LengthX"
  Bus Creator3/1 -> Bus Creator2/10  "Box3D"
  Constant17/1 -> Bus Creator2/13  "measConfidence"
  py/1 -> Bus Creator2/5  "py"
  Constant36/1 -> Bus Creator7/4  "px"
  Constant16/1 -> Bus Creator2/12  "ClassificationScore"
  Constant42/1 -> Bus Creator7/14  "StationaryFlag"
  SensorData/1 -> Assignment/1
  px/1 -> Bus Creator2/4  "px"
  Constant39/1 -> Bus Creator7/7  "vy"
  Constant35/1 -> Bus Creator7/1  "TimeStamp"
  Constant38/1 -> Bus Creator7/6  "vx"
  TIME_STAMP/1 -> Bus Creator2/1  "TimeStamp"
  Switch/1 -> Assignment/2
  iter/1 -> Assignment/3
  Bus Creator6/1 -> Bus Creator7/10  "Box3D"
  Constant10/1 -> Bus Creator1/2  "RefY"
  NOISE_COV/1 -> Bus Creator2/8  "NoiseCovarience"
  Constant21/1 -> Bus Creator3/4  "LengthX"
  Constant1/1 -> Bus Creator4/2  "RefY"
  Constant25/1 -> Bus Creator6/2  "RefY"
  Constant26/1 -> Bus Creator6/3  "RefZ"
  Constant29/1 -> Bus Creator6/6  "LengthZ"
  Constant30/1 -> Bus Creator4/1  "RefX"
  vx/1 -> Bus Creator2/6  "vx"
  Constant13/1 -> Bus Creator2/14  "StationaryFlag"
  Constant22/1 -> Bus Creator3/5  "LengthY"
  Constant24/1 -> Bus Creator6/1  "RefX"
  Constant40/1 -> Bus Creator7/3  "cameraID"
  Constant28/1 -> Bus Creator6/5  "LengthY"
  Assignment/1 -> C1/1
  Constant15/1 -> Bus Creator7/11  "Classification"
  Constant14/1 -> Bus Creator2/3  "cameraID"
  vy/1 -> Bus Creator2/7  "vy"
  OBJ_TYPE/1 -> Bus Creator2/11  "Classification"

== system Fusion_Frame_Model_Architecture/SENSOR_MEASUREMENTS/RADAR_CAMERA_EGO_SENSOR_INTERFACE/CameraSensors/Camera2/ExtractMeasParam1 ==
  idx : Inport
  time : Inport  Port=2
  Constant : Constant  Value=CAM2_PX
  Constant1 : Constant  Value=CAM2_PY
  Constant2 : Constant  Value=CAM2_VX
  Constant3 : Constant  Value=CAM2_VY
  Constant4 : Constant  Value=CAM2_objClassID
  Constant5 : Constant  Value=CAM2_MeasNoise
  Constant6 : Constant  Value=CAM2_detTimeStamp
  Data Type Conversion : DataTypeConversion  OutDataTypeStr=int16
  MeasNoise : Selector  NumberOfDimensions=4  InputPortWidth=3  IndexOptions=Index vector (port),Select all,Select all,Index vector (port)  Indices=[1 3],1,1,1  OutputSizes=1,1,1,1
  PosX : Selector  NumberOfDimensions=2  InputPortWidth=3  IndexOptions=Index vector (port),Index vector (port)  Indices=[1 3],1  OutputSizes=1,1
  PosY : Selector  NumberOfDimensions=2  InputPortWidth=3  IndexOptions=Index vector (port),Index vector (port)  Indices=[1 3],1  OutputSizes=1,1
  Reshape : Reshape  OutputDimensionality=Customize  OutputDimensions=[4,4]
  VelX : Selector  NumberOfDimensions=2  InputPortWidth=3  IndexOptions=Index vector (port),Index vector (port)  Indices=[1 3],1  OutputSizes=1,1
  VelY : Selector  NumberOfDimensions=2  InputPortWidth=3  IndexOptions=Index vector (port),Index vector (port)  Indices=[1 3],1  OutputSizes=1,1
  snr : Selector  NumberOfDimensions=2  InputPortWidth=3  IndexOptions=Index vector (port),Index vector (port)  Indices=[1 3],1  OutputSizes=1,1
  timeStamp : Selector  NumberOfDimensions=2  InputPortWidth=3  IndexOptions=Select all,Index vector (port)  Indices=[1 3],1  OutputSizes=1,1
  PX : Outport
  PY : Outport  Port=2
  VX : Outport  Port=3
  VY : Outport  Port=4
  OBJ_TYPE : Outport  Port=5
  NOISE_COV : Outport  Port=6
  measCaptureTime : Outport  Port=7
  wires:
  Constant3/1 -> VelY/1
  Constant2/1 -> VelX/1
  VelY/1 -> VY/1
  Constant/1 -> PosX/1
  idx/1 -> MeasNoise/3, snr/3, VelY/3, VelX/3, PosY/3, PosX/3
  Constant1/1 -> PosY/1
  VelX/1 -> VX/1
  PosX/1 -> PX/1
  PosY/1 -> PY/1
  time/1 -> timeStamp/2, MeasNoise/2, snr/2, VelY/2, VelX/2, PosY/2, PosX/2
  Constant4/1 -> snr/1
  snr/1 -> Data Type Conversion/1
  Constant5/1 -> MeasNoise/1
  Constant6/1 -> timeStamp/1
  MeasNoise/1 -> Reshape/1
  timeStamp/1 -> measCaptureTime/1
  Reshape/1 -> NOISE_COV/1
  Data Type Conversion/1 -> OBJ_TYPE/1

== system Fusion_Frame_Model_Architecture/SENSOR_MEASUREMENTS/RADAR_CAMERA_EGO_SENSOR_INTERFACE/CameraSensors/Camera2/IsValid2 ==
  idx : Inport
  px : Inport  Port=2
  py : Inport  Port=3
  vx : Inport  Port=4
  vy : Inport  Port=5
  Abs{,1..3} (4 alike) : Abs
  Add : Sum  Inputs=++++
  Constant : Constant  Value=uint16(0)
  Data Type Conversion : DataTypeConversion  OutDataTypeStr=uint16
  Switch : Switch  Threshold=0.0001
  ID : Outport
  wires:
  Add/1 -> Switch/2
  Abs2/1 -> Add/3
  Constant/1 -> Switch/3
  Abs/1 -> Add/1
  px/1 -> Abs/1
  Abs3/1 -> Add/4
  Abs1/1 -> Add/2
  vy/1 -> Abs3/1
  py/1 -> Abs1/1
  vx/1 -> Abs2/1
  idx/1 -> Data Type Conversion/1
  Switch/1 -> ID/1
  Data Type Conversion/1 -> Switch/1

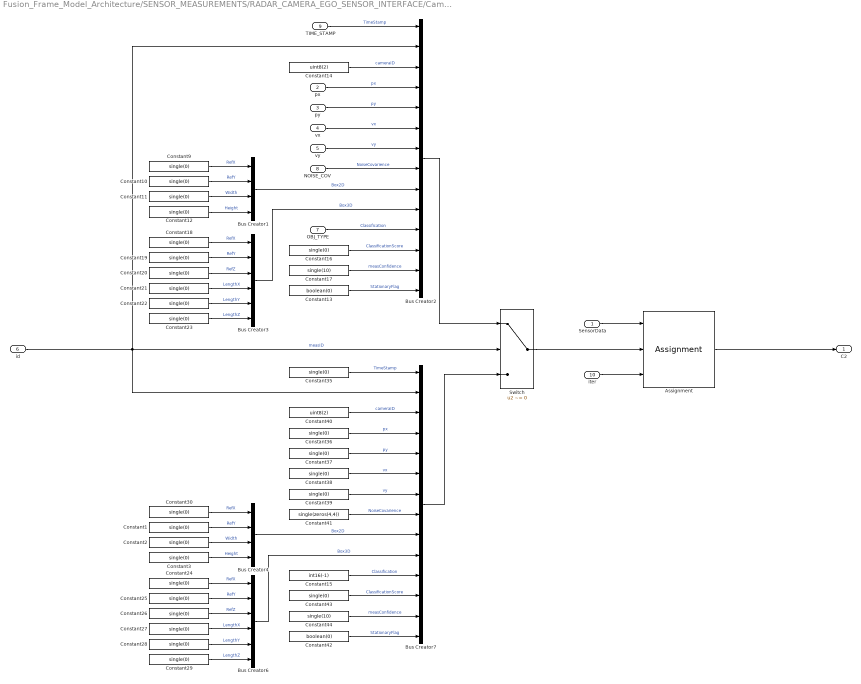
== system Fusion_Frame_Model_Architecture/SENSOR_MEASUREMENTS/RADAR_CAMERA_EGO_SENSOR_INTERFACE/CameraSensors/Camera2/Subsystem1 ==
  SensorData : Inport
  px : Inport  Port=2
  py : Inport  Port=3
  vx : Inport  Port=4
  vy : Inport  Port=5
  id : Inport  Port=6
  OBJ_TYPE : Inport  Port=7
  NOISE_COV : Inport  Port=8
  TIME_STAMP : Inport  Port=9
  iter : Inport  Port=10
  Assignment : Assignment  DiagnosticForDimensions=Warning  IndexOptions=Index vector (port)  Indices=1  OutputSizes=1
  Bus Creator1 : BusCreator  Inputs=4  OutDataTypeStr=Bus: BoxParam2D  NonVirtualBus=on
  Bus Creator2 : BusCreator  Inputs=14  OutDataTypeStr=Bus: CameraMeasParam  NonVirtualBus=on
  Bus Creator3 : BusCreator  Inputs=6  OutDataTypeStr=Bus: BoxParam3D  NonVirtualBus=on
  Bus Creator4 : BusCreator  Inputs=4  OutDataTypeStr=Bus: BoxParam2D  NonVirtualBus=on
  Bus Creator6 : BusCreator  Inputs=6  OutDataTypeStr=Bus: BoxParam3D  NonVirtualBus=on
  Bus Creator7 : BusCreator  Inputs=14  OutDataTypeStr=Bus: CameraMeasParam  NonVirtualBus=on
  Constant{1..3,9..12,16,18..30,35..39,43} (27 alike) : Constant  Value=single(0)
  Constant13 : Constant  Value=boolean(0)
  Constant14 : Constant  Value=uint8(2)
  Constant15 : Constant  Value=int16(-1)
  Constant17 : Constant  Value=single(10)
  Constant40 : Constant  Value=uint8(2)
  Constant41 : Constant  Value=single(zeros(4,4))
  Constant42 : Constant  Value=boolean(0)
  Constant44 : Constant  Value=single(10)
  Switch : Switch  Criteria=u2 ~= 0
  C2 : Outport
  wires:
  Bus Creator4/1 -> Bus Creator7/9  "Box2D"
  Bus Creator1/1 -> Bus Creator2/9  "Box2D"
  Bus Creator7/1 -> Switch/3
  Constant3/1 -> Bus Creator4/4  "Height"
  Constant44/1 -> Bus Creator7/13  "measConfidence"
  Constant19/1 -> Bus Creator3/2  "RefY"
  id/1 -> Bus Creator7/2, Bus Creator2/2, Switch/2  "measID"
  Bus Creator2/1 -> Switch/1
  Constant2/1 -> Bus Creator4/3  "Width"
  Constant12/1 -> Bus Creator1/4  "Height"
  Constant43/1 -> Bus Creator7/12  "ClassificationScore"
  Constant41/1 -> Bus Creator7/8  "NoiseCovarience"
  Constant20/1 -> Bus Creator3/3  "RefZ"
  Constant37/1 -> Bus Creator7/5  "py"
  Constant23/1 -> Bus Creator3/6  "LengthZ"
  Constant11/1 -> Bus Creator1/3  "Width"
  Constant18/1 -> Bus Creator3/1  "RefX"
  Constant9/1 -> Bus Creator1/1  "RefX"
  Constant27/1 -> Bus Creator6/4  "LengthX"
  Bus Creator3/1 -> Bus Creator2/10  "Box3D"
  Constant17/1 -> Bus Creator2/13  "measConfidence"
  py/1 -> Bus Creator2/5  "py"
  Constant36/1 -> Bus Creator7/4  "px"
  Constant16/1 -> Bus Creator2/12  "ClassificationScore"
  Constant42/1 -> Bus Creator7/14  "StationaryFlag"
  SensorData/1 -> Assignment/1
  px/1 -> Bus Creator2/4  "px"
  Constant39/1 -> Bus Creator7/7  "vy"
  Constant35/1 -> Bus Creator7/1  "TimeStamp"
  Constant38/1 -> Bus Creator7/6  "vx"
  TIME_STAMP/1 -> Bus Creator2/1  "TimeStamp"
  Switch/1 -> Assignment/2
  iter/1 -> Assignment/3
  Bus Creator6/1 -> Bus Creator7/10  "Box3D"
  Constant10/1 -> Bus Creator1/2  "RefY"
  NOISE_COV/1 -> Bus Creator2/8  "NoiseCovarience"
  Constant21/1 -> Bus Creator3/4  "LengthX"
  Constant1/1 -> Bus Creator4/2  "RefY"
  Constant25/1 -> Bus Creator6/2  "RefY"
  Constant26/1 -> Bus Creator6/3  "RefZ"
  Constant29/1 -> Bus Creator6/6  "LengthZ"
  Constant30/1 -> Bus Creator4/1  "RefX"
  vx/1 -> Bus Creator2/6  "vx"
  Constant13/1 -> Bus Creator2/14  "StationaryFlag"
  Constant22/1 -> Bus Creator3/5  "LengthY"
  Constant24/1 -> Bus Creator6/1  "RefX"
  Constant40/1 -> Bus Creator7/3  "cameraID"
  Constant28/1 -> Bus Creator6/5  "LengthY"
  Assignment/1 -> C2/1
  Constant15/1 -> Bus Creator7/11  "Classification"
  Constant14/1 -> Bus Creator2/3  "cameraID"
  vy/1 -> Bus Creator2/7  "vy"
  OBJ_TYPE/1 -> Bus Creator2/11  "Classification"

== system Fusion_Frame_Model_Architecture/SENSOR_MEASUREMENTS/RADAR_CAMERA_EGO_SENSOR_INTERFACE/CameraSensors/Camera3/ExtractMeasParam1 ==
  idx : Inport
  time : Inport  Port=2
  Constant : Constant  Value=CAM3_PX
  Constant1 : Constant  Value=CAM3_PY
  Constant2 : Constant  Value=CAM3_VX
  Constant3 : Constant  Value=CAM3_VY
  Constant4 : Constant  Value=CAM3_objClassID
  Constant5 : Constant  Value=CAM3_MeasNoise
  Constant6 : Constant  Value=CAM3_detTimeStamp
  Data Type Conversion : DataTypeConversion  OutDataTypeStr=int16
  MeasNoise : Selector  NumberOfDimensions=4  InputPortWidth=3  IndexOptions=Index vector (port),Select all,Select all,Index vector (port)  Indices=[1 3],1,1,1  OutputSizes=1,1,1,1
  PosX : Selector  NumberOfDimensions=2  InputPortWidth=3  IndexOptions=Index vector (port),Index vector (port)  Indices=[1 3],1  OutputSizes=1,1
  PosY : Selector  NumberOfDimensions=2  InputPortWidth=3  IndexOptions=Index vector (port),Index vector (port)  Indices=[1 3],1  OutputSizes=1,1
  Reshape : Reshape  OutputDimensionality=Customize  OutputDimensions=[4,4]
  VelX : Selector  NumberOfDimensions=2  InputPortWidth=3  IndexOptions=Index vector (port),Index vector (port)  Indices=[1 3],1  OutputSizes=1,1
  VelY : Selector  NumberOfDimensions=2  InputPortWidth=3  IndexOptions=Index vector (port),Index vector (port)  Indices=[1 3],1  OutputSizes=1,1
  snr : Selector  NumberOfDimensions=2  InputPortWidth=3  IndexOptions=Index vector (port),Index vector (port)  Indices=[1 3],1  OutputSizes=1,1
  timeStamp : Selector  NumberOfDimensions=2  InputPortWidth=3  IndexOptions=Select all,Index vector (port)  Indices=[1 3],1  OutputSizes=1,1
  PX : Outport
  PY : Outport  Port=2
  VX : Outport  Port=3
  VY : Outport  Port=4
  OBJ_TYPE : Outport  Port=5
  NOISE_COV : Outport  Port=6
  measCaptureTime : Outport  Port=7
  wires:
  Constant3/1 -> VelY/1
  Constant2/1 -> VelX/1
  VelY/1 -> VY/1
  Constant/1 -> PosX/1
  idx/1 -> MeasNoise/3, snr/3, VelY/3, VelX/3, PosY/3, PosX/3
  Constant1/1 -> PosY/1
  VelX/1 -> VX/1
  PosX/1 -> PX/1
  PosY/1 -> PY/1
  time/1 -> timeStamp/2, MeasNoise/2, snr/2, VelY/2, VelX/2, PosY/2, PosX/2
  Constant4/1 -> snr/1
  snr/1 -> Data Type Conversion/1
  Constant5/1 -> MeasNoise/1
  Constant6/1 -> timeStamp/1
  MeasNoise/1 -> Reshape/1
  timeStamp/1 -> measCaptureTime/1
  Reshape/1 -> NOISE_COV/1
  Data Type Conversion/1 -> OBJ_TYPE/1

== system Fusion_Frame_Model_Architecture/SENSOR_MEASUREMENTS/RADAR_CAMERA_EGO_SENSOR_INTERFACE/CameraSensors/Camera3/IsValid2 ==
  idx : Inport
  px : Inport  Port=2
  py : Inport  Port=3
  vx : Inport  Port=4
  vy : Inport  Port=5
  Abs{,1..3} (4 alike) : Abs
  Add : Sum  Inputs=++++
  Constant : Constant  Value=uint16(0)
  Data Type Conversion : DataTypeConversion  OutDataTypeStr=uint16
  Switch : Switch  Threshold=0.0001
  ID : Outport
  wires:
  Add/1 -> Switch/2
  Abs2/1 -> Add/3
  Constant/1 -> Switch/3
  Abs/1 -> Add/1
  px/1 -> Abs/1
  Abs3/1 -> Add/4
  Abs1/1 -> Add/2
  vy/1 -> Abs3/1
  py/1 -> Abs1/1
  vx/1 -> Abs2/1
  idx/1 -> Data Type Conversion/1
  Switch/1 -> ID/1
  Data Type Conversion/1 -> Switch/1

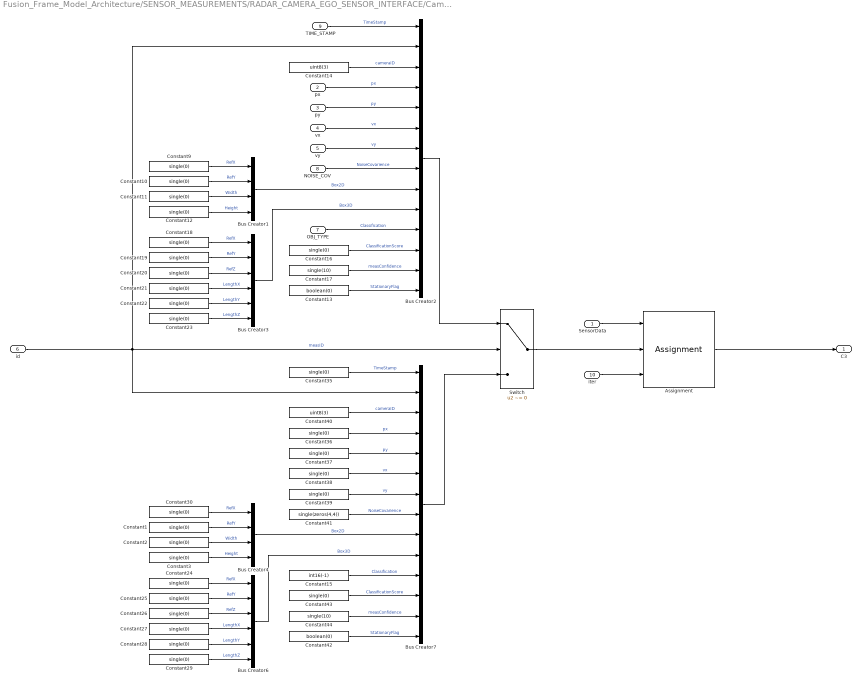
== system Fusion_Frame_Model_Architecture/SENSOR_MEASUREMENTS/RADAR_CAMERA_EGO_SENSOR_INTERFACE/CameraSensors/Camera3/Subsystem1 ==
  SensorData : Inport
  px : Inport  Port=2
  py : Inport  Port=3
  vx : Inport  Port=4
  vy : Inport  Port=5
  id : Inport  Port=6
  OBJ_TYPE : Inport  Port=7
  NOISE_COV : Inport  Port=8
  TIME_STAMP : Inport  Port=9
  iter : Inport  Port=10
  Assignment : Assignment  DiagnosticForDimensions=Warning  IndexOptions=Index vector (port)  Indices=1  OutputSizes=1
  Bus Creator1 : BusCreator  Inputs=4  OutDataTypeStr=Bus: BoxParam2D  NonVirtualBus=on
  Bus Creator2 : BusCreator  Inputs=14  OutDataTypeStr=Bus: CameraMeasParam  NonVirtualBus=on
  Bus Creator3 : BusCreator  Inputs=6  OutDataTypeStr=Bus: BoxParam3D  NonVirtualBus=on
  Bus Creator4 : BusCreator  Inputs=4  OutDataTypeStr=Bus: BoxParam2D  NonVirtualBus=on
  Bus Creator6 : BusCreator  Inputs=6  OutDataTypeStr=Bus: BoxParam3D  NonVirtualBus=on
  Bus Creator7 : BusCreator  Inputs=14  OutDataTypeStr=Bus: CameraMeasParam  NonVirtualBus=on
  Constant{1..3,9..12,16,18..30,35..39,43} (27 alike) : Constant  Value=single(0)
  Constant13 : Constant  Value=boolean(0)
  Constant14 : Constant  Value=uint8(3)
  Constant15 : Constant  Value=int16(-1)
  Constant17 : Constant  Value=single(10)
  Constant40 : Constant  Value=uint8(3)
  Constant41 : Constant  Value=single(zeros(4,4))
  Constant42 : Constant  Value=boolean(0)
  Constant44 : Constant  Value=single(10)
  Switch : Switch  Criteria=u2 ~= 0
  C3 : Outport
  wires:
  Bus Creator4/1 -> Bus Creator7/9  "Box2D"
  Bus Creator1/1 -> Bus Creator2/9  "Box2D"
  Bus Creator7/1 -> Switch/3
  Constant3/1 -> Bus Creator4/4  "Height"
  Constant44/1 -> Bus Creator7/13  "measConfidence"
  Constant19/1 -> Bus Creator3/2  "RefY"
  id/1 -> Bus Creator7/2, Bus Creator2/2, Switch/2  "measID"
  Bus Creator2/1 -> Switch/1
  Constant2/1 -> Bus Creator4/3  "Width"
  Constant12/1 -> Bus Creator1/4  "Height"
  Constant43/1 -> Bus Creator7/12  "ClassificationScore"
  Constant41/1 -> Bus Creator7/8  "NoiseCovarience"
  Constant20/1 -> Bus Creator3/3  "RefZ"
  Constant37/1 -> Bus Creator7/5  "py"
  Constant23/1 -> Bus Creator3/6  "LengthZ"
  Constant11/1 -> Bus Creator1/3  "Width"
  Constant18/1 -> Bus Creator3/1  "RefX"
  Constant9/1 -> Bus Creator1/1  "RefX"
  Constant27/1 -> Bus Creator6/4  "LengthX"
  Bus Creator3/1 -> Bus Creator2/10  "Box3D"
  Constant17/1 -> Bus Creator2/13  "measConfidence"
  py/1 -> Bus Creator2/5  "py"
  Constant36/1 -> Bus Creator7/4  "px"
  Constant16/1 -> Bus Creator2/12  "ClassificationScore"
  Constant42/1 -> Bus Creator7/14  "StationaryFlag"
  SensorData/1 -> Assignment/1
  px/1 -> Bus Creator2/4  "px"
  Constant39/1 -> Bus Creator7/7  "vy"
  Constant35/1 -> Bus Creator7/1  "TimeStamp"
  Constant38/1 -> Bus Creator7/6  "vx"
  TIME_STAMP/1 -> Bus Creator2/1  "TimeStamp"
  Switch/1 -> Assignment/2
  iter/1 -> Assignment/3
  Bus Creator6/1 -> Bus Creator7/10  "Box3D"
  Constant10/1 -> Bus Creator1/2  "RefY"
  NOISE_COV/1 -> Bus Creator2/8  "NoiseCovarience"
  Constant21/1 -> Bus Creator3/4  "LengthX"
  Constant1/1 -> Bus Creator4/2  "RefY"
  Constant25/1 -> Bus Creator6/2  "RefY"
  Constant26/1 -> Bus Creator6/3  "RefZ"
  Constant29/1 -> Bus Creator6/6  "LengthZ"
  Constant30/1 -> Bus Creator4/1  "RefX"
  vx/1 -> Bus Creator2/6  "vx"
  Constant13/1 -> Bus Creator2/14  "StationaryFlag"
  Constant22/1 -> Bus Creator3/5  "LengthY"
  Constant24/1 -> Bus Creator6/1  "RefX"
  Constant40/1 -> Bus Creator7/3  "cameraID"
  Constant28/1 -> Bus Creator6/5  "LengthY"
  Assignment/1 -> C3/1
  Constant15/1 -> Bus Creator7/11  "Classification"
  Constant14/1 -> Bus Creator2/3  "cameraID"
  vy/1 -> Bus Creator2/7  "vy"
  OBJ_TYPE/1 -> Bus Creator2/11  "Classification"
